simulink library "mpclib"  (Simulink 7.4)
settings: Solver=ode45  SolverMode=SingleTasking  StartTime=0.0  StopTime=10.0  RelTol=1e-3
libraries: mpclib x1, simulink x1
settings Model: Creator=jowen  LastModifiedBy=rchen

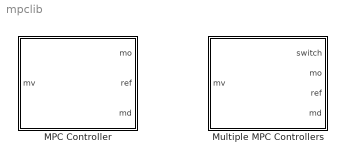
== system mpclib ==
  MPC Controller : Subsystem  InitFcn=mpc_init  StartFcn=mpc_chkdimensions_sim  mask(MPC){mpcobj=, n_mv=0, x0=[], ref_from_ws=off, ref_signal_name=[], ref_preview=on, md_from_ws=off, md_signal_name=[], md_preview=on, from_project=off, md_inport=on, mv_inport=off, lims_inport=off, switch_inport=off, enable_value=0, project_file=MPCtask.mat, project_name=, task_name=, is_multiple=0}
      mask prompts: mpcobj "MPC Object"; n_mv "Starting Number of MVs"; x0 "Initial Extended State"; ref_from_ws "Reference from Workspace"; ref_signal_name "Reference"; ref_preview "Reference Preview"; md_from_ws "Measured Disturbance from workspace"; md_signal_name "Measured Disturbance"; md_preview "Measured Disturbance Preview"; from_project "Controller From Project"; md_inport "MD Signal"; mv_inport "External MV Signal"; lims_inport "External Limits"; switch_inport "External Switching Signal for Optimization"; enable_value "Value enabling optimization"; project_file "Project File"; project_name "Project Name"; task_name "Task Name"; is_multiple "Flag indicating the block is part of multiple blocks"
      mask init:
      | [ts,A,Cm,Dvm,Bu,Bv,PTYPE,nu,nv,nym,ny,nx,degrees,L,MuKduINV,KduINV,Kx,Ku1,Kut,Kr,Kv,zmin,rhsc0,Mlim,Mx,Mu1,Mv,rhsa0,TAB,optimalseq,utarget,lastx,lastu,p,Jm,DUFree,uoff,yoff,voff,myoff,no_md,no_ref,ref_from_ws,ref_signal,ref_preview,md_from_ws,md_signal,md_preview,maxiter,nxQP,openloopflag,md_inport,no_ym,mv_inport,no_mv,wtab,lims_inport,no_umin,no_umax,no_ymin,no_ymax,switch_inport,no_switch,enable_value,is_multiple] = mpc_get_param_sim;
      | mpc_block_resize(gcb);
      settings: DeleteFcn=mpc_deletetask  OpenFcn=mpc_mask
      mask Display:
      | fprintf('MPC');
      | port_label('output', 1, 'mv')
      | port_label('input', 1, 'mo')
      | port_label('input', 2, 'ref')
      | port_label('input', 3, 'md')
  Multiple MPC Controllers : Subsystem  StartFcn=mpc_chkdimensions_sim_multiple  mask(Multiple MPC){Nmpc=1, theMPC=1, md_inport_multiple=on, mv_inport_multiple=off, lims_inport_multiple=off, mpcobjs={''}, x0s={'[]'}, ref_signal_name_multiple=[], ref_preview_multiple=on, ref_from_ws_multiple=off, md_signal_name_multiple=[], md_preview_multiple=on, md_from_ws_multiple=off, nmv=0, linswitch=0}
      mask prompts: Nmpc "Number of multiple MPC controllers"; theMPC "Currently selected MPC controller"; md_inport_multiple "External MD Signal"; mv_inport_multiple "External MV Signal"; lims_inport_multiple "External Limits"; mpcobjs "MPC objects"; x0s "MPC initial states"; ref_signal_name_multiple "Reference signal"; ref_preview_multiple "Reference preview flag"; ref_from_ws_multiple "Reference from Workspace"; md_signal_name_multiple "Measured disturbance signal"; md_preview_multiple "Measured disturbance preview flag"; md_from_ws_multiple "Measured disturbance from workspace"; nmv "Number of MVs"; linswitch "Linearization Switch"
      mask init:
      | mpc_block_resize_multiple(gcb)
      settings: DeleteFcn=mpc_deletetask_multiple  OpenFcn=mpc_mask_multiple
      mask Display:
      | fprintf('Multiple\nMPC');
      | port_label('output', 1, 'mv')
      | port_label('input', 1, 'switch')
      | port_label('input', 2, 'mo')
      | port_label('input', 3, 'ref')
      | port_label('input', 4, 'md')

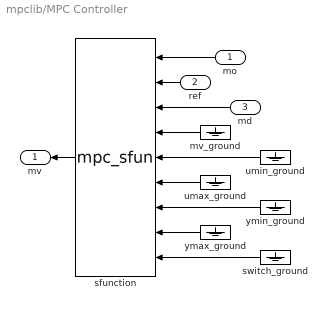
== system mpclib/MPC Controller ==
  mo : Inport  OutDataType=sfix(16)  OutScaling=2^0
  ref : Inport  Port=2  OutDataType=sfix(16)  OutScaling=2^0
  md : Inport  Port=3  OutDataType=sfix(16)  OutScaling=2^0
  mv_ground : Ground
  sfunction : S-Function  FunctionName=mpc_sfun  Parameters=ts,A,Cm,Dvm,Bu,Bv,PTYPE,nu,nv,nym,ny,nx,degrees,L,MuKduINV,KduINV,Kx,Ku1,Kut,Kr,Kv,zmin,rhsc0,Mlim,Mx,Mu1,Mv,rhsa0,TAB,optimalseq,utarget,lastx,lastu,p,Jm,DUFree,uoff,yoff,voff,myoff,no_md,no_ref,ref_from_ws,ref_signal,ref_preview,md_from_ws,md_signal,md_preview,maxiter,nxQP,openloopflag,md_inport,no_ym,mv_inport,no_mv,wtab,lims_inport,no_umin,no_umax,no_ymin,no_ymax,switch_inport,no_switch,enable_value,is_multiple  EnableBusSupport=off
  switch_ground : Ground
  umax_ground : Ground
  umin_ground : Ground
  ymax_ground : Ground
  ymin_ground : Ground
  mv : Outport  OutDataType=sfix(16)  OutScaling=2^0
  wires:
  mo/1 -> sfunction/1
  sfunction/1 -> mv/1
  ref/1 -> sfunction/2
  md/1 -> sfunction/3
  mv_ground/1 -> sfunction/4
  umin_ground/1 -> sfunction/5
  umax_ground/1 -> sfunction/6
  ymin_ground/1 -> sfunction/7
  ymax_ground/1 -> sfunction/8
  switch_ground/1 -> sfunction/9

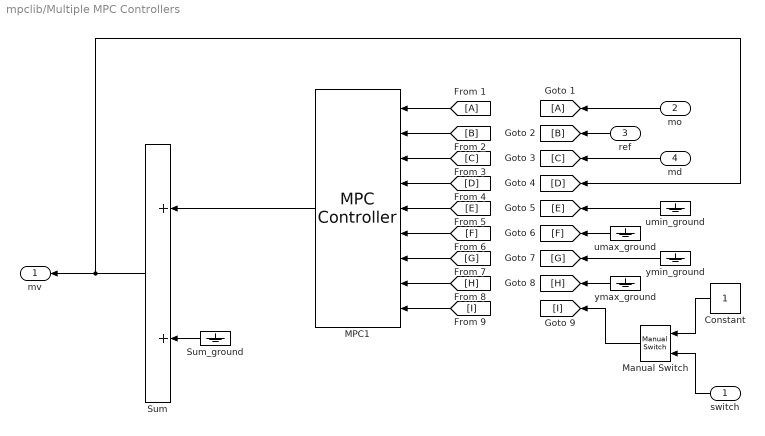
== system mpclib/Multiple MPC Controllers ==
  switch : Inport  OutDataType=sfix(16)  OutScaling=2^0
  mo : Inport  Port=2  OutDataType=sfix(16)  OutScaling=2^0
  ref : Inport  Port=3  OutDataType=sfix(16)  OutScaling=2^0
  md : Inport  Port=4  OutDataType=sfix(16)  OutScaling=2^0
  Constant : Constant  OutDataType=sfix(16)  OutScaling=2^0
  MPC1 : mpclib/MPC Controller  SystemSampleTime=-1  n_mv=0  x0=[]  ref_from_ws=off  ref_signal_name=[]  ref_preview=on  md_from_ws=off  md_signal_name=[]  md_preview=on  from_project=off  md_inport=on  mv_inport=on  lims_inport=on  switch_inport=on  enable_value=1  project_file=MPCtask.mat  is_multiple=1
  Manual Switch : simulink/Signal Routing/Manual Switch  SystemSampleTime=-1  sw=0  action=0  varsize=off
  Sum : Sum  OutDataType=sfix(16)  OutScaling=2^0
  Sum_ground : Ground
  umax_ground : Ground
  umin_ground : Ground
  ymax_ground : Ground
  ymin_ground : Ground
  mv : Outport  OutDataType=sfix(16)  OutScaling=2^0
  wires:
  [I] -> MPC1/9
  [H] -> MPC1/8
  [G] -> MPC1/7
  [F] -> MPC1/6
  [E] -> MPC1/5
  [D] -> MPC1/4
  [C] -> MPC1/3
  [B] -> MPC1/2
  [A] -> MPC1/1
  ref/1 -> [B]
  mo/1 -> [A]
  Sum/1 -> mv/1, [D]
  MPC1/1 -> Sum/1
  md/1 -> [C]
  umin_ground/1 -> [E]
  umax_ground/1 -> [F]
  ymin_ground/1 -> [G]
  ymax_ground/1 -> [H]
  Sum_ground/1 -> Sum/2
  Manual Switch/1 -> [I]
  switch/1 -> Manual Switch/2
  Constant/1 -> Manual Switch/1
